simulink model "pump_3"  (R2018b)
settings: Solver=ode45  StartTime=0.0  StopTime=210  MaxStep=0.1  RelTol=1e-3  EnableMultiTasking=on
undefined symbols (not defined in the file): path_carnot
libraries: carnot x6, simulink x1
settings Model: Creator=drhf  LastModifiedBy=drhf
settings DataIOCC: LimitDataPoints=on  SaveFormat=Array
settings OptimizationCC: ExpressionDepthLimit=2147483647  LifeSpan=inf
settings DebuggingCC: UnderspecifiedInitializationDetection=Classic  MergeDetectMultiDrivingBlocksExec=none  SolverPrmCheckMsg=warning  StateNameClashWarn=warning  SFUnexpectedBacktrackingDiag=warning  SFNoUnconditionalDefaultTransitionDiag=warning  SFExecutionAtInitializationDiag=none
settings HardwareCC: ProdBitPerPointer=32  ProdBitPerSizeT=32  ProdBitPerPtrDiffT=32  ProdLargestAtomicFloat=None  ProdIntDivRoundTo=Undefined  ProdEndianess=Unspecified  ProdWordSize=32  ProdHWDeviceType=32-bit Generic
settings ModelReferenceCC: PropagateSignalLabelsOutOfModel=off
settings SFSimCC: SimUseLocalCustomCode=off
settings RTWCC: RTWUseLocalCustomCode=off
settings CodeAppCC: StateflowObjectComments=on
settings GRTTargetCC: TargetLangStandard=C89/C90 (ANSI)  GeneratePreprocessorConditionals=Disable all  CombineOutputUpdateFcns=off  GRTInterface=on
settings ConfigComp: CovMetricSettings=dw  CovHtmlReporting=on  CovSaveCumulativeToWorkspaceVar=on  CovSaveSingleToWorkspaceVar=on  CovExternalEMLEnable=off

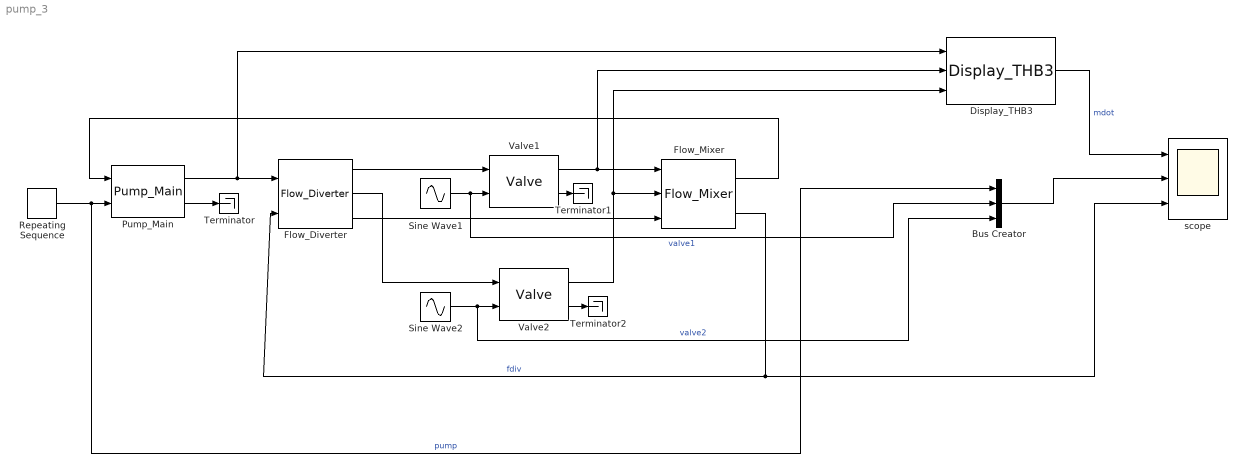
== system pump_3 ==
  Bus Creator : BusCreator  Inputs=3
  Display_THB3 : carnot/Outputs/Display_THB3  t=off  m=on  p=off  id=off  mix=off  d=off
  Flow_Diverter : carnot/Hydraulics/Flow_Diverter
  Flow_Mixer : carnot/Hydraulics/Flow_Mixer
  Pump_Main : carnot/Hydraulics/Pump_Main  Tini=20  p0=3e5  IDpreset=pressure drop  fluid=Water  mix=0  mix2=0  mix3=0  t1=5  PathName=fullfile(path_carnot('libsl'), 'Hydraulics', 'Pump_Main', 'parameter_set')  FileName='Pump6m.mat'  userPath=off  userParam=off  a0=60000  a1=-43200  a2=0  dia=0.025  UA=1  mcp=4182  e0=50  e1=28.8  e2=-10.368
  Repeating Sequence : simulink/Sources/Repeating Sequence  rep_seq_t=[0 20 60 200]  rep_seq_y=[0 0 1 1]
  Sine Wave1 : Sin  Amplitude=0.6  Bias=0.5  Frequency=1/20  SampleTime=0
  Sine Wave2 : Sin  Amplitude=0.6  Bias=0.5  Frequency=1/20  Phase=pi  SampleTime=0
  Terminator : Terminator
  Terminator1 : Terminator
  Terminator2 : Terminator
  Valve1 : carnot/Hydraulics/Valve  vtyp=linear  psi_0=0.04  kvs=1.6  dt_V=30
  Valve2 : carnot/Hydraulics/Valve  vtyp=linear  psi_0=0.04  kvs=1.6  dt_V=30
  scope : Scope  NumInputPorts=3
  wires:
  Repeating Sequence/1 -> Pump_Main/2, Bus Creator/1  "pump"
  Pump_Main/2 -> Terminator/1
  Sine Wave1/1 -> Bus Creator/2, Valve1/2  "valve1"
  Pump_Main/1 -> Display_THB3/1, Flow_Diverter/1
  Flow_Diverter/1 -> Valve1/1
  Sine Wave2/1 -> Bus Creator/3, Valve2/2  "valve2"
  Flow_Diverter/2 -> Valve2/1
  Flow_Diverter/3 -> Flow_Mixer/3
  Flow_Mixer/2 -> scope/3, Flow_Diverter/2  "fdiv"
  Flow_Mixer/1 -> Pump_Main/1
  Display_THB3/1 -> scope/1  "mdot"
  Bus Creator/1 -> scope/2
  Valve1/1 -> Display_THB3/2, Flow_Mixer/1
  Valve2/1 -> Display_THB3/3, Flow_Mixer/2
  Valve1/2 -> Terminator1/1
  Valve2/2 -> Terminator2/1
